simulink model "blockdemo"  (Simulink 6.3)
settings: Solver=VariableStepDiscrete  StartTime=0  StopTime=2^8  RelTol=1e-3
InitFcn:
  | %% DSPBuilder Start
  | alt_dspbuilder_update_model(bdroot)
  | %% DSPBuilder End
libraries: allblocks_alteradspbuilder2 x11, simulink x1
settings Model: Creator=mjervis  LastModifiedBy=delphick
settings DataIOCC: SignalLoggingName=sigsOut
settings OptimizationCC: BlockReduction=off  BooleanDataType=off  InlineInvariantSignals=on
settings DebuggingCC: SolverPrmCheckMsg=none
settings HardwareCC: TargetUnknown=on

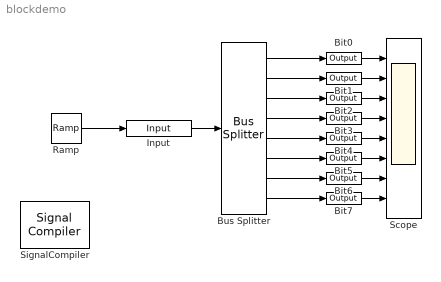
== system blockdemo ==
  Bit0 : allblocks_alteradspbuilder2/Output  iofile=C:\workspace_clean\Documentation\DesignExamples\Tutorials\UnitBlocks\IOBus\BusSplitter\tb_blockdemo\blockdemo_Bit0.capture  BusType=Single Bit  bwl=8  bwr=0  PORTTYPE=Output
  Bit1 : allblocks_alteradspbuilder2/Output  iofile=C:\workspace_clean\Documentation\DesignExamples\Tutorials\UnitBlocks\IOBus\BusSplitter\tb_blockdemo\blockdemo_Bit1.capture  BusType=Single Bit  bwl=8  bwr=0  PORTTYPE=Output
  Bit2 : allblocks_alteradspbuilder2/Output  iofile=C:\workspace_clean\Documentation\DesignExamples\Tutorials\UnitBlocks\IOBus\BusSplitter\tb_blockdemo\blockdemo_Bit2.capture  BusType=Single Bit  bwl=8  bwr=0  PORTTYPE=Output
  Bit3 : allblocks_alteradspbuilder2/Output  iofile=C:\workspace_clean\Documentation\DesignExamples\Tutorials\UnitBlocks\IOBus\BusSplitter\tb_blockdemo\blockdemo_Bit3.capture  BusType=Single Bit  bwl=8  bwr=0  PORTTYPE=Output
  Bit4 : allblocks_alteradspbuilder2/Output  iofile=C:\workspace_clean\Documentation\DesignExamples\Tutorials\UnitBlocks\IOBus\BusSplitter\tb_blockdemo\blockdemo_Bit4.capture  BusType=Single Bit  bwl=8  bwr=0  PORTTYPE=Output
  Bit5 : allblocks_alteradspbuilder2/Output  iofile=C:\workspace_clean\Documentation\DesignExamples\Tutorials\UnitBlocks\IOBus\BusSplitter\tb_blockdemo\blockdemo_Bit5.capture  BusType=Single Bit  bwl=8  bwr=0  PORTTYPE=Output
  Bit6 : allblocks_alteradspbuilder2/Output  iofile=C:\workspace_clean\Documentation\DesignExamples\Tutorials\UnitBlocks\IOBus\BusSplitter\tb_blockdemo\blockdemo_Bit6.capture  BusType=Single Bit  bwl=8  bwr=0  PORTTYPE=Output
  Bit7 : allblocks_alteradspbuilder2/Output  iofile=C:\workspace_clean\Documentation\DesignExamples\Tutorials\UnitBlocks\IOBus\BusSplitter\tb_blockdemo\blockdemo_Bit7.capture  BusType=Single Bit  bwl=8  bwr=0  PORTTYPE=Output
  Bus Splitter : allblocks_alteradspbuilder2/Bus Splitter  BusType=Signed Integer  bwl=8  bwr=0
  Input : allblocks_alteradspbuilder2/Input  iofile=C:\workspace_clean\Documentation\DesignExamples\Tutorials\UnitBlocks\IOBus\BusSplitter\tb_blockdemo\blockdemo_Input.salt  BusType=Unsigned Integer  bwl=8  bwr=0  SpecifyClock=off  PORTTYPE=Input
      settings: AttributesFormatString=%<BusType>
  Ramp : simulink/Sources/Ramp  slope=1  start=0  X0=0
  Scope : Scope  NumInputPorts=8
      settings: TimeRange=256  YMin=-0.5~-0.5~-0.5~-0.5~-0.5~-0.5~-0.5~-0.5  YMax=1.5~1.5~1.5~1.5~1.5~1.5~1.5~1.5  SampleInput=on  SampleTime=1
  SignalCompiler : allblocks_alteradspbuilder2/Signal Compiler  DeviceFamily=Stratix IV  DeviceName=AUTO  EnableSignalTap=off  SignalTapDepth=128  UseBoardBlock=off  StpUseDefaultClock=on  StpClock=clock
  wires:
  Bus Splitter/1 -> Bit0/1
  Bus Splitter/2 -> Bit1/1
  Bus Splitter/3 -> Bit2/1
  Bus Splitter/4 -> Bit3/1
  Bus Splitter/5 -> Bit4/1
  Bus Splitter/6 -> Bit5/1
  Bus Splitter/7 -> Bit6/1
  Bus Splitter/8 -> Bit7/1
  Input/1 -> Bus Splitter/1
  Ramp/1 -> Input/1
  Bit0/1 -> Scope/1
  Bit1/1 -> Scope/2
  Bit2/1 -> Scope/3
  Bit3/1 -> Scope/4
  Bit4/1 -> Scope/5
  Bit5/1 -> Scope/6
  Bit6/1 -> Scope/7
  Bit7/1 -> Scope/8
